simulink model "ECS_FOS"  (Simulink 8.2)
settings: Solver=ode45  StartTime=0.0  StopTime=18000  RelTol=1e-3
InitFcn:
  | load('loss_coeff_mixing_junction.mat')
  | load('SampleOutput.mat')
  | load('HydProp.mat')
  | load('HydraulicLoad.mat')
  | load('initavload.mat')
  | load('SampleFuelBurn.mat')
values from neighbouring files (symbols this model uses):
  FuelBurn = [0 0 0 0 0 0 0 0 0 0 0 0 ... (18249 elements, 1x18249)]    [Benchmark_data1.mat]
  fueltankdata =     [Benchmark_data1.mat]
undefined symbols (not defined in the file or in its folder): AirProp, F1, F2, HUGHES_TREITLER, magnitude, PN_70147, PumpProp
libraries: PowerFlowLib x46, simulink x4
(part 5 of 5)

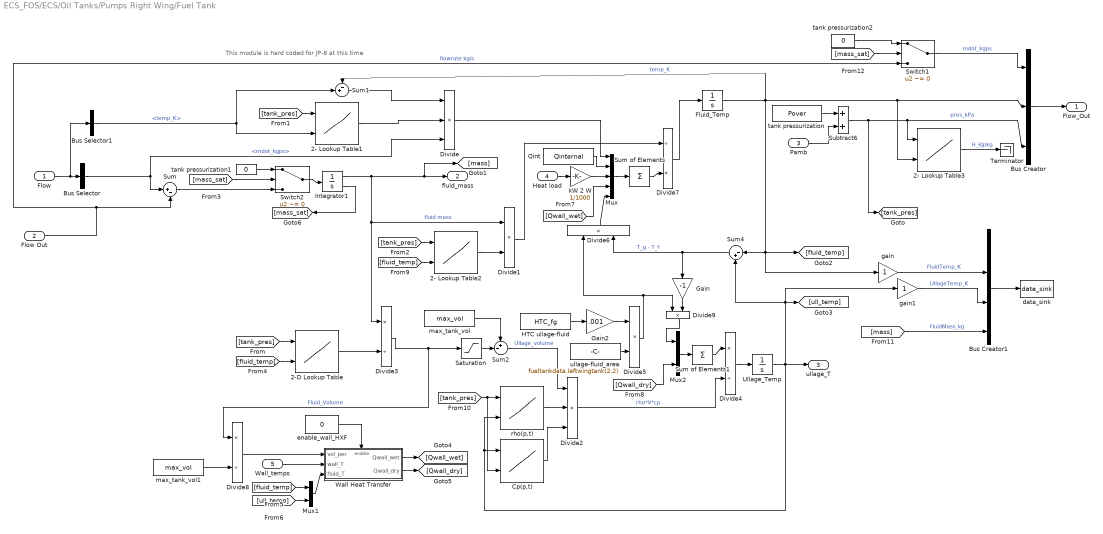
== system ECS_FOS/ECS/Oil Tanks/Pumps Right Wing/Fuel Tank ==
  note: This module is hard coded for JP-8 at this time
  Flow : Inport
  Flow Out : Inport  Port=2
  Pamb : Inport  Port=3
  Heat load : Inport  Port=4
  Wall_temps : Inport  Port=5
  2- Lookup Table1 : Lookup_n-D  BreakpointsForDimension1=F1.P  BreakpointsForDimension2=F1.T  Table=F1.Cp_pt  RndMeth=Simplest  InputSameDT=on
  2- Lookup Table2 : Lookup_n-D  BreakpointsForDimension1=F1.P  BreakpointsForDimension2=F1.T  Table=F1.Cp_pt  RndMeth=Simplest  InputSameDT=on
  2- Lookup Table3 : Lookup_n-D  BreakpointsForDimension1=F1.P  BreakpointsForDimension2=F1.T  Table=F1.H_pt  RndMeth=Simplest  InputSameDT=on
  2-D Lookup Table : Lookup_n-D  BreakpointsForDimension1=F1.P  BreakpointsForDimension2=F1.T  Table=F1.Rho_pt  RndMeth=Simplest  InputSameDT=on
  Bus Creator : BusCreator  Inputs=3
  Bus Creator1 : BusCreator
  Bus Selector : BusSelector  OutputSignals=mdot_kgps
  Bus Selector1 : BusSelector  OutputSignals=temp_K
  Cp(p,t) : Lookup_n-D  BreakpointsForDimension1=AirProp.P  BreakpointsForDimension2=AirProp.T  Table=AirProp.Cp_pt  RndMeth=Simplest  InputSameDT=on
  Divide : Product  Inputs=***
  Divide{1,5..6,9} (4 alike) : Product  Inputs=**
  Divide2 : Product  Inputs=***
  Divide3 : Product  Inputs=*/
  Divide4 : Product  Inputs=*/
  Divide7 : Product  Inputs=/*
  Divide8 : Product  Inputs=*/
  Fluid_Temp : Integrator  InitialCondition=fld_Tint + 273.15  LimitOutput=on  UpperSaturationLimit=800  LowerSaturationLimit=eps
  Gain : Gain  Gain=-1
  Gain2 : Gain  Gain=.001
  HTC ullage-fluid : Constant  Value=HTC_fg
  Integrator1 : Integrator  InitialCondition=m_init  LimitOutput=on  LowerSaturationLimit=1  ShowSaturationPort=on
  Mux : Mux  Inputs=5
  Mux1 : Mux  Inputs=2
  Mux2 : Mux  Inputs=2
  Qint : Constant  Value=Qinternal
  Saturation : Saturate  UpperLimit=inf  LowerLimit=eps  ZeroCross=off
  Subtract6 : Sum
  Sum : Sum  Inputs=|+-
  Sum of Elements : Sum  Inputs=+
  Sum of Elements1 : Sum  Inputs=+
  Sum1 : Sum  Inputs=-+|
  Sum2 : Sum  Inputs=+-|
  Sum4 : Sum  Inputs=|-+
  Switch1 : Switch  Criteria=u2 ~= 0  Threshold=-1
  Switch2 : Switch  Criteria=u2 ~= 0  Threshold=-1
  Terminator : Terminator
  Ullage_Temp : Integrator  InitialCondition=ull_Tint + 273.15  LimitOutput=on  LowerSaturationLimit=eps
  Wall Heat Transfer : Subsystem  TreatAsAtomicUnit=on
  data_sink : PowerFlowLib/Support Functions//Tools/data_sink
      link override global_data_goto: GotoTag=gdata_PowerFlowLibEnergyPowerSystemsThermalFuelFuelTank
  enable_wall_HXF : Constant  Value=0
  gain : Gain
  gain1 : Gain
  kW 2 W : Gain  Gain=1/1000
  max_tank_vol : Constant  Value=max_vol
  max_tank_vol1 : Constant  Value=max_vol
  rho(p,t) : Lookup_n-D  BreakpointsForDimension1=AirProp.P  BreakpointsForDimension2=AirProp.T  Table=AirProp.Rho_pt  RndMeth=Simplest  InputSameDT=on
  tank pressurization : Constant  Value=Pover
  tank pressurization1 : Constant  Value=0
  tank pressurization2 : Constant  Value=0
  ullage-fluid_area : Constant  Value=fueltankdata.leftwingtank(2,2)
  Flow_Out : Outport
  fluid_mass : Outport  Port=2
  ullage_T : Outport  Port=3
  wires:
  Switch2/1 -> Integrator1/1
  tank pressurization1/1 -> Switch2/1
  [mass_sat] -> Switch2/2
  Integrator1/2 -> [mass_sat]
  Sum/1 -> Switch2/3
  tank pressurization2/1 -> Switch1/1
  [mass_sat] -> Switch1/2
  [mass] -> Bus Creator1/4  "FluidMass_kg"
  gain1/1 -> Bus Creator1/3  "UllageTemp_K"
  gain/1 -> Bus Creator1/2  "FluidTemp_K"
  Bus Creator1/1 -> data_sink/1
  kW 2 W/1 -> Mux/3
  2- Lookup Table3/1 -> Terminator/1  "H_kJpkg"
  Flow/1 -> Bus Selector/1, Bus Selector1/1
  Bus Selector/1 -> Divide/3, Sum/1  "<mdot_kgps>"
  Flow Out/1 -> Sum/2, Switch1/3  "flowrate kg/s"
  Integrator1/1 -> fluid_mass/1, [mass], Divide3/1, Divide1/1  "fluid mass"
  Bus Selector1/1 -> Sum1/2, 2- Lookup Table1/2  "<temp_K>"
  Sum1/1 -> Divide/1
  2- Lookup Table2/1 -> Divide1/2
  rho(p,t)/1 -> Divide2/2
  Cp(p,t)/1 -> Divide2/3
  Divide3/1 -> Saturation/1, Divide8/1  "Fluid_Volume"
  max_tank_vol/1 -> Sum2/1
  Sum2/1 -> Divide2/1  "Ullage_volume"
  Divide4/1 -> Ullage_Temp/1
  Ullage_Temp/1 -> ullage_T/1, gain1/1, Sum4/2, [ull_temp], rho(p,t)/2, Cp(p,t)/1
  Fluid_Temp/1 -> 2- Lookup Table3/2, Bus Creator/2, Sum1/1, gain/1, Sum4/1, [fluid_temp]  "temp_K"
  HTC ullage-fluid/1 -> Gain2/1
  ullage-fluid_area/1 -> Divide5/2
  Sum4/1 -> Divide6/2, Gain/1  "T_g - T_f"
  Divide1/1 -> Divide7/1
  Divide7/1 -> Fluid_Temp/1
  Divide5/1 -> Divide6/1, Divide9/1
  Pamb/1 -> Subtract6/2
  tank pressurization/1 -> Subtract6/1
  Subtract6/1 -> 2- Lookup Table3/1, Bus Creator/3, [tank_pres]  "pres_kPa"
  Bus Creator/1 -> Flow_Out/1
  Saturation/1 -> Sum2/2
  [tank_pres] -> 2-D Lookup Table/1
  2-D Lookup Table/1 -> Divide3/2
  [tank_pres] -> 2- Lookup Table1/1
  2- Lookup Table1/1 -> Divide/2
  [tank_pres] -> 2- Lookup Table2/1
  max_tank_vol1/1 -> Divide8/2
  Switch1/1 -> Bus Creator/1  "mdot_kgps"
  Divide/1 -> Mux/1
  Qint/1 -> Mux/2
  Heat load/1 -> kW 2 W/1
  Sum of Elements/1 -> Divide7/2
  Mux/1 -> Sum of Elements/1
  [fluid_temp] -> 2-D Lookup Table/2
  Divide8/1 -> Wall Heat Transfer/1(vol_per)
  Wall_temps/1 -> Wall Heat Transfer/2(wall_T)
  [fluid_temp] -> Mux1/1
  [ull_temp] -> Mux1/2
  Mux1/1 -> Wall Heat Transfer/3(fluid_T)
  Wall Heat Transfer/1(Qwall_wet) -> [Qwall_wet]
  Wall Heat Transfer/2(Qwall_dry) -> [Qwall_dry]
  Divide6/1 -> Mux/5
  Divide2/1 -> Divide4/2  "rho*V*cp"
  Mux2/1 -> Sum of Elements1/1
  Sum of Elements1/1 -> Divide4/1
  Gain/1 -> Divide9/2
  Divide9/1 -> Mux2/1
  [Qwall_dry] -> Mux2/2
  [Qwall_wet] -> Mux/4
  [fluid_temp] -> 2- Lookup Table2/2
  enable_wall_HXF/1 -> Wall Heat Transfer/Enable
  Gain2/1 -> Divide5/1
  [tank_pres] -> rho(p,t)/1, Cp(p,t)/2

== system ECS_FOS/ECS/Right PACK/Distribution of bleed air ==
  Bleed to Valve : Inport
  Bleed to ACM : Inport  Port=2
  bleed_temp : Inport  Port=3
  bleed_pres : Inport  Port=4
  Bus Creator1 : BusCreator  Inputs=3
  Bus Creator2 : BusCreator  Inputs=3
  Scope : Scope  NumInputPorts=4
      settings: YMin=0~386.7~110~0.2  YMax=0.055~387.8~160~0.85  SaveName=ScopeData42  SampleInput=on  SampleTime=1
  Flow to Mix Junc. : Outport
  Flow to HX : Outport  Port=2
  wires:
  Bleed to ACM/1 -> Bus Creator2/1, Scope/4  "mdot_kgps"
  bleed_temp/1 -> Bus Creator2/2, Bus Creator1/2, Scope/2
  bleed_pres/1 -> Bus Creator2/3, Bus Creator1/3, Scope/3
  Bleed to Valve/1 -> Bus Creator1/1, Scope/1  "mdot_kgps"
  Bus Creator1/1 -> Flow to Mix Junc./1
  Bus Creator2/1 -> Flow to HX/1

== system ECS_FOS/ECS/Right PACK/Ram air inlet ==
  Temp_amb : Inport
  Temp_comp : Inport  Port=2
  2 : Constant  Value=T_35
  Bus Creator : BusCreator  Inputs=3
  Bus Selector4 : BusSelector  OutputSignals=temp_K
  Constant1 : Constant  Value=22.5
  Gain : Gain  Gain=0.95
  Gain1 : Gain
  Memory : Memory  X0=ram_air
  Subtract : Sum  Inputs=+-
  Switch : Switch  Criteria=u2 ~= 0  Threshold=30
  Flow Out : Outport
  wires:
  Temp_comp/1 -> Bus Selector4/1
  Bus Selector4/1 -> Subtract/1  "<temp_K>"
  2/1 -> Subtract/2
  Subtract/1 -> Switch/2
  Gain/1 -> Switch/3
  Switch/1 -> Memory/1
  Temp_amb/1 -> Bus Creator/1  "temp_K"
  Constant1/1 -> Bus Creator/2  "pres_kPa"
  Bus Creator/1 -> Flow Out/1
  Memory/1 -> Bus Creator/3, Gain1/1, Gain/1  "mdot_kgps"
  Gain1/1 -> Switch/1

== system ECS_FOS/ECS/Right PACK/Subsystem1 ==
  Bypass Ratio : Inport
  Air from PHX : Inport  Port=2
  Bus Creator : BusCreator  Inputs=3
  Bus Creator1 : BusCreator  Inputs=3
  Bus Selector : BusSelector  OutputSignals=mdot_kgps,temp_K,pres_kPa
  Fcn1 : Fcn  Expr=1-u(1)
  Gain : Gain
  Gain1 : Gain
  Gain2 : Gain
  Product : Product  RndMeth=Zero
  Product1 : Product  RndMeth=Zero
  Saturation : Saturate  UpperLimit=inf  LowerLimit=eps
  Air to Mix Junc : Outport
  Air to Comp : Outport  Port=2
  wires:
  Gain1/1 -> Bus Creator1/2  "temp_K"
  Gain/1 -> Bus Creator1/3  "pres_kPa"
  Bus Creator1/1 -> Air to Mix Junc/1
  Bus Selector/3 -> Gain/1, Gain2/1  "<pres_kPa>"
  Product1/1 -> Bus Creator1/1  "mdot_kgps"
  Saturation/1 -> Bus Creator/1  "mdot_kgps"
  Bus Selector/2 -> Gain1/1, Bus Creator/2  "<temp_K>"
  Bus Creator/1 -> Air to Comp/1
  Bus Selector/1 -> Product/2, Product1/1  "<mdot_kgps>"
  Air from PHX/1 -> Bus Selector/1
  Product/1 -> Saturation/1
  Bypass Ratio/1 -> Fcn1/1, Product1/2
  Fcn1/1 -> Product/1
  Gain2/1 -> Bus Creator/3  "pres_kPa"

== system ECS_FOS/ECS/Right PACK/User-set_ supply_pressure ==
  Flow In : Inport
  Cabin Pres. : Inport  Port=2
  Bus Creator4 : BusCreator  Inputs=3
  Bus Selector3 : BusSelector  OutputSignals=mdot_kgps,temp_K
  Gain1 : Gain  Gain=1.1
  Flow Out : Outport
  wires:
  Bus Selector3/1 -> Bus Creator4/1  "<mdot_kgps>"
  Bus Selector3/2 -> Bus Creator4/2  "<temp_K>"
  Gain1/1 -> Bus Creator4/3  "pres_kPa"
  Flow In/1 -> Bus Selector3/1
  Bus Creator4/1 -> Flow Out/1
  Cabin Pres./1 -> Gain1/1

== system ECS_FOS/ECS/Right PACK/Valve1 ==
  Flow In : Inport
  Bus Creator2 : BusCreator  Inputs=3
  Bus Selector2 : BusSelector  OutputSignals=mdot_kgps,pres_kPa,temp_K
  Math Functin : Math  Operator=pow  SaturateOnIntegerOverflow=on
  Product : Product  RndMeth=Zero
  Sum : Sum  Inputs=|-+
  "Value?? -- MAW" : Constant  Value=50
  get u : Gain
  mass_flow_rate1 : Constant  Value=2
  Flow Out : Outport
  wires:
  Bus Creator2/1 -> Flow Out/1
  Flow In/1 -> Bus Selector2/1
  Bus Selector2/1 -> Bus Creator2/1, get u/1  "<mdot_kgps>"
  get u/1 -> Math Functin/1
  mass_flow_rate1/1 -> Math Functin/2
  Math Functin/1 -> Product/2
  Product/1 -> Sum/1
  Bus Selector2/2 -> Sum/2  "<pres_kPa>"
  Sum/1 -> Bus Creator2/2  "pres_kPa"
  Bus Selector2/3 -> Bus Creator2/3  "<temp_K>"
  "Value?? -- MAW"/1 -> Product/1

== system ECS_FOS/ECS/Thermal_sources_from Electrical_power_model1/ThermalSource ==
  LoadBus : BusCreator  Inputs=1
  Load : Outport
  wires:
  LoadBus/1 -> Load/1

== system ECS_FOS/ECS/Thermal_sources_from Electrical_power_model1/ThermalSource3 ==
  LoadBus : BusCreator  Inputs=1
  Load : Outport
  wires:
  LoadBus/1 -> Load/1

== system ECS_FOS/ECS/Thermal_sources_from Electrical_power_model1/ThermalSource4 ==
  LoadBus : BusCreator  Inputs=1
  Load : Outport
  wires:
  LoadBus/1 -> Load/1

== system ECS_FOS/ECS/Thermal_sources_from Electrical_power_model1/ThermalSource5 ==
  LoadBus : BusCreator  Inputs=1
  Load : Outport
  wires:
  LoadBus/1 -> Load/1

== system ECS_FOS/ECS/Cabin Zone/Cabin Temperature/Fuselage_parameters1 ==
  Area_fuselage_total_m2 : Constant  Value=A_fuselage
  Bus Creator : BusCreator  Inputs=2
  Coating_resistance_ m2KpW : Product  Inputs=*/
  Coating_thermal_ conductivity_WpmK : Constant  Value=K_coating
  Coating_thickness_m : Constant  Value=L_coating
  Display : Display
  Inside_HTC_Wpm2K : Constant  Value=h_inside
  Inside_convection_ resistance_m2KpW : Product  Inputs=*/
  Insulation_resistance_ m2KpW : Product  Inputs=*/
  Insulation_thermal_ conductivity_WpmK : Constant  Value=K_insulation
  Insulation_thickness_m : Constant  Value=L_insulation
  Outside_HTC_Wpm2K1 : Constant  Value=h_outside
  Outside_convection_ resistance_m2KpW : Product  Inputs=*/
  Overall_HTC_based_on_ any_fuselage_area_Wpm2K : Product  Inputs=*/
  Shell_resistance_ m2KpW : Product  Inputs=*/
  Shell_thermal_ conductivity_WpmK : Constant  Value=K_shell
  Shell_thickness_m : Constant  Value=L_shell
  Total_resistance_ m2KpW : Sum  Inputs=+++++
  constant_unity : Constant
  constant_unity1 : Constant
  constant_unity2 : Constant
  Fuselage Parameters : Outport
  wires:
  Overall_HTC_based_on_ any_fuselage_area_Wpm2K/1 -> Bus Creator/2, Display/1  "U_Wpm2K"
  Bus Creator/1 -> Fuselage Parameters/1
  constant_unity/1 -> Outside_convection_ resistance_m2KpW/1
  Outside_HTC_Wpm2K1/1 -> Outside_convection_ resistance_m2KpW/2
  Shell_thickness_m/1 -> Shell_resistance_ m2KpW/1
  Shell_thermal_ conductivity_WpmK/1 -> Shell_resistance_ m2KpW/2
  Insulation_thickness_m/1 -> Insulation_resistance_ m2KpW/1
  Insulation_thermal_ conductivity_WpmK/1 -> Insulation_resistance_ m2KpW/2
  Coating_thickness_m/1 -> Coating_resistance_ m2KpW/1
  Coating_thermal_ conductivity_WpmK/1 -> Coating_resistance_ m2KpW/2
  constant_unity1/1 -> Inside_convection_ resistance_m2KpW/1
  Inside_HTC_Wpm2K/1 -> Inside_convection_ resistance_m2KpW/2
  Outside_convection_ resistance_m2KpW/1 -> Total_resistance_ m2KpW/1
  Shell_resistance_ m2KpW/1 -> Total_resistance_ m2KpW/2
  Insulation_resistance_ m2KpW/1 -> Total_resistance_ m2KpW/3
  Coating_resistance_ m2KpW/1 -> Total_resistance_ m2KpW/4
  Inside_convection_ resistance_m2KpW/1 -> Total_resistance_ m2KpW/5
  constant_unity2/1 -> Overall_HTC_based_on_ any_fuselage_area_Wpm2K/1
  Total_resistance_ m2KpW/1 -> Overall_HTC_based_on_ any_fuselage_area_Wpm2K/2
  Area_fuselage_total_m2/1 -> Bus Creator/1  "area_m2"

== system ECS_FOS/ECS/Cabin Zone/Cabin Temperature/Kinetic Heating ==
  note: PLEASE note that that the correlation for the recovery temperature
      | is gives in "Aircraft Systems", by Ian Moir and Allan Seabridge,
      | 3rd edition, pp 260
  Amb. Temp. K : Inport
  Mach# : Inport  Port=2
  Bias : Bias  Bias=1
  Gain : Gain  Gain=0.18
  Math Function1 : Math  Operator=magnitude^2  SaturateOnIntegerOverflow=on
  Product1 : Product  RndMeth=Zero
  Recovery Temp [K] : Outport
  wires:
  Mach#/1 -> Math Function1/1
  Product1/1 -> Recovery Temp [K]/1
  Amb. Temp. K/1 -> Product1/1
  Bias/1 -> Product1/2
  Gain/1 -> Bias/1
  Math Function1/1 -> Gain/1

== system ECS_FOS/ECS/FOHX Left Wing/HX_Calcs/Fluid 1 Heat Transfer Calculation ==
  note: NTU calculation
  note: Secondary Fluid heat transfer coefficient
  note: It calculates the outlet temperature and enthalpy.
  Inputs : Inport
  2-D Lookup Table : Lookup_n-D  BreakpointsForDimension1=F1.P  BreakpointsForDimension2=F1.T  Table=F1.H_pt  RndMeth=Simplest  InputSameDT=on
  2-D Lookup Table1 : Lookup_n-D  BreakpointsForDimension1=F1.P  BreakpointsForDimension2=F1.T  Table=F1.H_pt  RndMeth=Simplest  InputSameDT=on
  2-D Lookup Table2 : Lookup_n-D  BreakpointsForDimension1=F1.P  BreakpointsForDimension2=F1.T  Table=F1.H_pt  RndMeth=Simplest  InputSameDT=on
  2-D Lookup Table3 : Lookup_n-D  BreakpointsForDimension1=F1.P  BreakpointsForDimension2=F1.T  Table=F1.Cp_pt  RndMeth=Simplest  InputSameDT=on
  Bus Selector : BusSelector  OutputSignals=mdot1_in,T1_in,P1_in
  Constant : Constant  Value=0
  Constant10 : Constant  Value=A1_c
  Constant2 : Constant  Value=N1
  Constant4 : Constant
  Constant8 : Constant  Value=N1
  Constant9 : Constant  Value=A1_s*2
  Fcn6 : Fcn  Expr=u(2) + (u(1)-u(2))*u(3)
  Gain1 : Gain  Gain=-1
  Gain3 : Gain
  HTC Calc : Subsystem
  Math Function3 : Math  SaturateOnIntegerOverflow=on
  Mux4 : Mux  Inputs=3
  Product2 : Product  Inputs=***//  RndMeth=Zero
  Product6 : Product  Inputs=***/  RndMeth=Zero
  Subtract2 : Sum  Inputs=+-
  kJ/kg to J/kg : Gain  Gain=1000
  h_out_h : Outport
  T_out_h : Outport  Port=2
  q_h : Outport  Port=3
  wires:
  [T_out] -> 2-D Lookup Table1/2
  [T_in] -> 2-D Lookup Table/2
  2-D Lookup Table/1 -> Subtract2/1
  2-D Lookup Table1/1 -> Subtract2/2
  2-D Lookup Table2/1 -> h_out_h/1
  Product6/1 -> Gain1/1
  Constant4/1 -> Product6/2
  [mdot_in] -> Product6/1
  Subtract2/1 -> Product6/3
  Fcn6/1 -> T_out_h/1, [T_out], 2-D Lookup Table2/2  "T_out"
  Mux4/1 -> Fcn6/1
  [e2NTU1] -> Mux4/3
  Constant/1 -> Mux4/2
  Gain1/1 -> q_h/1
  Constant2/1 -> Product6/4
  Product2/1 -> Gain3/1  "NTU"
  Constant9/1 -> Product2/2
  [alpha] -> Product2/1
  Constant8/1 -> Product2/3
  HTC Calc/1(alpha_a) -> [alpha]
  [T_in] -> HTC Calc/3(T_a)
  Constant10/1 -> HTC Calc/2(A_ca)
  [mdot_in] -> HTC Calc/1(mdot_a)
  [T_in] -> 2-D Lookup Table3/2
  2-D Lookup Table3/1 -> kJ/kg to J/kg/1
  Inputs/1 -> Bus Selector/1
  Bus Selector/1 -> [mdot_in]  "<mdot1_in>"
  Bus Selector/2 -> [T_in]  "<T1_in>"
  Bus Selector/3 -> [P_in]  "<P1_in>"
  Math Function3/1 -> [e2NTU1]
  Gain3/1 -> Math Function3/1
  [mdot_in] -> Product2/4
  [cp] -> Product2/5
  [T_in] -> Mux4/1
  [P_in] -> 2-D Lookup Table/1
  [P_in] -> 2-D Lookup Table1/1
  [P_in] -> 2-D Lookup Table2/1
  [P_in] -> 2-D Lookup Table3/1
  kJ/kg to J/kg/1 -> [cp]

== system ECS_FOS/ECS/FOHX Left Wing/HX_Calcs/Fluid 2 Heat Transfer Calculation ==
  note: NTU calculation
  note: Secondary Fluid heat transfer coefficient
  note: It calculates the outlet temperature and enthalpy.
  Inputs : Inport
  1-D Lookup Table : Lookup_n-D  NumberOfTableDimensions=1  BreakpointsForDimension1=F2.T  Table=F2.cp_T  RndMeth=Simplest  InputSameDT=on
  1-D Lookup Table1 : Lookup_n-D  NumberOfTableDimensions=1  BreakpointsForDimension1=F2.T  Table=F2.H  RndMeth=Simplest  InputSameDT=on
  1-D Lookup Table2 : Lookup_n-D  NumberOfTableDimensions=1  BreakpointsForDimension1=F2.T  Table=F2.H  RndMeth=Simplest  InputSameDT=on
  1-D Lookup Table3 : Lookup_n-D  NumberOfTableDimensions=1  BreakpointsForDimension1=F2.T  Table=F2.H  RndMeth=Simplest  InputSameDT=on
  Bus Selector : BusSelector  OutputSignals=mdot2_in,T2_in,P2_in
  Constant : Constant  Value=0
  Constant10 : Constant  Value=A2_c
  Constant2 : Constant  Value=N2
  Constant4 : Constant
  Constant8 : Constant  Value=N2
  Constant9 : Constant  Value=A2_s*2
  Fcn6 : Fcn  Expr=u(2) + (u(1)-u(2))*u(3)
  Gain1 : Gain  Gain=-1
  Gain3 : Gain  Gain=-1
  HTC Calc : Subsystem
  Math Function3 : Math  SaturateOnIntegerOverflow=on
  Mux4 : Mux  Inputs=3
  Product2 : Product  Inputs=***//  RndMeth=Zero
  Product6 : Product  Inputs=***/  RndMeth=Zero
  Subtract2 : Sum  Inputs=+-
  Terminator : Terminator
  kJ/kg to J/kg : Gain  Gain=1000
  h_out : Outport
  T_out : Outport  Port=2
  q_h : Outport  Port=3
  wires:
  [T_out] -> 1-D Lookup Table3/1
  [T_in] -> 1-D Lookup Table2/1
  1-D Lookup Table2/1 -> Subtract2/1
  1-D Lookup Table3/1 -> Subtract2/2
  1-D Lookup Table1/1 -> h_out/1
  Product6/1 -> Gain1/1
  Constant4/1 -> Product6/2
  [mdot_in] -> Product6/1
  Subtract2/1 -> Product6/3
  Fcn6/1 -> [T_out], T_out/1, 1-D Lookup Table1/1  "T_out"
  Mux4/1 -> Fcn6/1
  [e2NTU1] -> Mux4/3
  Constant/1 -> Mux4/2
  Gain1/1 -> q_h/1
  Constant2/1 -> Product6/4
  Product2/1 -> Gain3/1  "NTU"
  Constant9/1 -> Product2/2
  [alpha] -> Product2/1
  Constant8/1 -> Product2/3
  HTC Calc/1(alpha_a) -> [alpha]
  [T_in] -> HTC Calc/3(T_a)
  Constant10/1 -> HTC Calc/2(A_ca)
  [mdot_in] -> HTC Calc/1(mdot_a)
  [T_in] -> 1-D Lookup Table/1
  1-D Lookup Table/1 -> kJ/kg to J/kg/1
  Inputs/1 -> Bus Selector/1
  Bus Selector/1 -> [mdot_in]  "<mdot2_in>"
  Bus Selector/2 -> [T_in]  "<T2_in>"
  Bus Selector/3 -> Terminator/1  "<P2_in>"
  Math Function3/1 -> [e2NTU1]
  Gain3/1 -> Math Function3/1
  [mdot_in] -> Product2/4
  [cp] -> Product2/5
  [T_in] -> Mux4/1
  kJ/kg to J/kg/1 -> [cp]

== system ECS_FOS/ECS/FOHX Left Wing/HX_Calcs/Input Processing ==
  Inputs : Inport
  Bus Creator : BusCreator  Inputs=6
  Bus Selector : BusSelector  OutputSignals=mdot1_in,P1_in,T1_in,mdot2_in,P2_in,T2_in
  Processed_Inputs : Outport
  wires:
  Bus Selector/1 -> Bus Creator/1  "<mdot1_in>"
  Bus Selector/2 -> Bus Creator/2  "<P1_in>"
  Bus Selector/3 -> Bus Creator/3  "<T1_in>"
  Bus Selector/4 -> Bus Creator/4  "<mdot2_in>"
  Bus Selector/5 -> Bus Creator/5  "<P2_in>"
  Bus Selector/6 -> Bus Creator/6  "<T2_in>"
  Inputs/1 -> Bus Selector/1  "Inputs"
  Bus Creator/1 -> Processed_Inputs/1

== system ECS_FOS/ECS/FOHX Right Wing/HX_Calcs/Fluid 1 Heat Transfer Calculation ==
  note: It calculates the outlet temperature and enthalpy.
  note: Secondary Fluid heat transfer coefficient
  note: NTU calculation
  Inputs : Inport
  2-D Lookup Table : Lookup_n-D  BreakpointsForDimension1=F1.P  BreakpointsForDimension2=F1.T  Table=F1.H_pt  RndMeth=Simplest  InputSameDT=on
  2-D Lookup Table1 : Lookup_n-D  BreakpointsForDimension1=F1.P  BreakpointsForDimension2=F1.T  Table=F1.H_pt  RndMeth=Simplest  InputSameDT=on
  2-D Lookup Table2 : Lookup_n-D  BreakpointsForDimension1=F1.P  BreakpointsForDimension2=F1.T  Table=F1.H_pt  RndMeth=Simplest  InputSameDT=on
  2-D Lookup Table3 : Lookup_n-D  BreakpointsForDimension1=F1.P  BreakpointsForDimension2=F1.T  Table=F1.Cp_pt  RndMeth=Simplest  InputSameDT=on
  Bus Selector : BusSelector  OutputSignals=mdot1_in,T1_in,P1_in
  Constant : Constant  Value=0
  Constant10 : Constant  Value=A1_c
  Constant2 : Constant  Value=N1
  Constant4 : Constant
  Constant8 : Constant  Value=N1
  Constant9 : Constant  Value=A1_s*2
  Fcn6 : Fcn  Expr=u(2) + (u(1)-u(2))*u(3)
  Gain1 : Gain  Gain=-1
  Gain3 : Gain
  HTC Calc : Subsystem
  Math Function3 : Math  SaturateOnIntegerOverflow=on
  Mux4 : Mux  Inputs=3
  Product2 : Product  Inputs=***//  RndMeth=Zero
  Product6 : Product  Inputs=***/  RndMeth=Zero
  Subtract2 : Sum  Inputs=+-
  kJ/kg to J/kg : Gain  Gain=1000
  h_out_h : Outport
  T_out_h : Outport  Port=2
  q_h : Outport  Port=3
  wires:
  kJ/kg to J/kg/1 -> [cp]
  [P_in] -> 2-D Lookup Table3/1
  [P_in] -> 2-D Lookup Table2/1
  [P_in] -> 2-D Lookup Table1/1
  [P_in] -> 2-D Lookup Table/1
  [T_in] -> Mux4/1
  [cp] -> Product2/5
  [mdot_in] -> Product2/4
  Gain3/1 -> Math Function3/1
  Math Function3/1 -> [e2NTU1]
  Bus Selector/3 -> [P_in]  "<P1_in>"
  Bus Selector/2 -> [T_in]  "<T1_in>"
  Bus Selector/1 -> [mdot_in]  "<mdot1_in>"
  Inputs/1 -> Bus Selector/1
  2-D Lookup Table3/1 -> kJ/kg to J/kg/1
  [T_in] -> 2-D Lookup Table3/2
  [mdot_in] -> HTC Calc/1(mdot_a)
  Constant10/1 -> HTC Calc/2(A_ca)
  [T_in] -> HTC Calc/3(T_a)
  HTC Calc/1(alpha_a) -> [alpha]
  Constant8/1 -> Product2/3
  [alpha] -> Product2/1
  Constant9/1 -> Product2/2
  Product2/1 -> Gain3/1  "NTU"
  Constant2/1 -> Product6/4
  Gain1/1 -> q_h/1
  Constant/1 -> Mux4/2
  [e2NTU1] -> Mux4/3
  Mux4/1 -> Fcn6/1
  Fcn6/1 -> 2-D Lookup Table2/2, [T_out], T_out_h/1  "T_out"
  Subtract2/1 -> Product6/3
  [mdot_in] -> Product6/1
  Constant4/1 -> Product6/2
  Product6/1 -> Gain1/1
  2-D Lookup Table2/1 -> h_out_h/1
  2-D Lookup Table1/1 -> Subtract2/2
  2-D Lookup Table/1 -> Subtract2/1
  [T_in] -> 2-D Lookup Table/2
  [T_out] -> 2-D Lookup Table1/2

== system ECS_FOS/ECS/FOHX Right Wing/HX_Calcs/Fluid 2 Heat Transfer Calculation ==
  note: It calculates the outlet temperature and enthalpy.
  note: Secondary Fluid heat transfer coefficient
  note: NTU calculation
  Inputs : Inport
  1-D Lookup Table : Lookup_n-D  NumberOfTableDimensions=1  BreakpointsForDimension1=F2.T  Table=F2.cp_T  RndMeth=Simplest  InputSameDT=on
  1-D Lookup Table1 : Lookup_n-D  NumberOfTableDimensions=1  BreakpointsForDimension1=F2.T  Table=F2.H  RndMeth=Simplest  InputSameDT=on
  1-D Lookup Table2 : Lookup_n-D  NumberOfTableDimensions=1  BreakpointsForDimension1=F2.T  Table=F2.H  RndMeth=Simplest  InputSameDT=on
  1-D Lookup Table3 : Lookup_n-D  NumberOfTableDimensions=1  BreakpointsForDimension1=F2.T  Table=F2.H  RndMeth=Simplest  InputSameDT=on
  Bus Selector : BusSelector  OutputSignals=mdot2_in,T2_in,P2_in
  Constant : Constant  Value=0
  Constant10 : Constant  Value=A2_c
  Constant2 : Constant  Value=N2
  Constant4 : Constant
  Constant8 : Constant  Value=N2
  Constant9 : Constant  Value=A2_s*2
  Fcn6 : Fcn  Expr=u(2) + (u(1)-u(2))*u(3)
  Gain1 : Gain  Gain=-1
  Gain3 : Gain  Gain=-1
  HTC Calc : Subsystem
  Math Function3 : Math  SaturateOnIntegerOverflow=on
  Mux4 : Mux  Inputs=3
  Product2 : Product  Inputs=***//  RndMeth=Zero
  Product6 : Product  Inputs=***/  RndMeth=Zero
  Subtract2 : Sum  Inputs=+-
  Terminator : Terminator
  kJ/kg to J/kg : Gain  Gain=1000
  h_out : Outport
  T_out : Outport  Port=2
  q_h : Outport  Port=3
  wires:
  kJ/kg to J/kg/1 -> [cp]
  [T_in] -> Mux4/1
  [cp] -> Product2/5
  [mdot_in] -> Product2/4
  Gain3/1 -> Math Function3/1
  Math Function3/1 -> [e2NTU1]
  Bus Selector/3 -> Terminator/1  "<P2_in>"
  Bus Selector/2 -> [T_in]  "<T2_in>"
  Bus Selector/1 -> [mdot_in]  "<mdot2_in>"
  Inputs/1 -> Bus Selector/1
  1-D Lookup Table/1 -> kJ/kg to J/kg/1
  [T_in] -> 1-D Lookup Table/1
  [mdot_in] -> HTC Calc/1(mdot_a)
  Constant10/1 -> HTC Calc/2(A_ca)
  [T_in] -> HTC Calc/3(T_a)
  HTC Calc/1(alpha_a) -> [alpha]
  Constant8/1 -> Product2/3
  [alpha] -> Product2/1
  Constant9/1 -> Product2/2
  Product2/1 -> Gain3/1  "NTU"
  Constant2/1 -> Product6/4
  Gain1/1 -> q_h/1
  Constant/1 -> Mux4/2
  [e2NTU1] -> Mux4/3
  Mux4/1 -> Fcn6/1
  Fcn6/1 -> 1-D Lookup Table1/1, T_out/1, [T_out]  "T_out"
  Subtract2/1 -> Product6/3
  [mdot_in] -> Product6/1
  Constant4/1 -> Product6/2
  Product6/1 -> Gain1/1
  1-D Lookup Table1/1 -> h_out/1
  1-D Lookup Table3/1 -> Subtract2/2
  1-D Lookup Table2/1 -> Subtract2/1
  [T_in] -> 1-D Lookup Table2/1
  [T_out] -> 1-D Lookup Table3/1

== system ECS_FOS/ECS/FOHX Right Wing/HX_Calcs/Input Processing ==
  Inputs : Inport
  Bus Creator : BusCreator  Inputs=6
  Bus Selector : BusSelector  OutputSignals=mdot1_in,P1_in,T1_in,mdot2_in,P2_in,T2_in
  Processed_Inputs : Outport
  wires:
  Bus Creator/1 -> Processed_Inputs/1
  Inputs/1 -> Bus Selector/1  "Inputs"
  Bus Selector/6 -> Bus Creator/6  "<T2_in>"
  Bus Selector/5 -> Bus Creator/5  "<P2_in>"
  Bus Selector/4 -> Bus Creator/4  "<mdot2_in>"
  Bus Selector/3 -> Bus Creator/3  "<T1_in>"
  Bus Selector/2 -> Bus Creator/2  "<P1_in>"
  Bus Selector/1 -> Bus Creator/1  "<mdot1_in>"

== system ECS_FOS/ECS/Fuel Tanks/Pumps/Center Fuel Tank/Wall Heat Transfer ==
  vol_per : Inport
  wall_T : Inport  Port=2
  fluid_T : Inport  Port=3
  Enable : EnablePort
  Abs : Abs
  Demux : Demux  Outputs=2
  Divide : Product  Inputs=**
  Divide1 : Product  Inputs=**
  Sum : Sum  Inputs=+-
  Sum1 : Sum  Inputs=-+
  Walls 1 to n : Constant  Value=1:size(fueltankdata.centertank,2)
  dry HTC : Gain  Gain=dryHTC
  total area : Bias  Bias=-[fueltankdata.centertank(11,:)]
  volume_% : Lookup_n-D  BreakpointsForDimension1=linspace(0,1,11)  BreakpointsForDimension2=linspace(1,6,6)  Table=fueltankdata.centertank  RndMeth=Simplest  InputSameDT=on
  wet HTC : Gain  Gain=wetHTC
  Qwall_wet : Outport
  Qwall_dry : Outport  Port=2
  wires:
  Walls 1 to n/1 -> volume_%/2
  vol_per/1 -> volume_%/1
  volume_%/1 -> total area/1, wet HTC/1  "wet area"
  fluid_T/1 -> Demux/1
  Demux/1 -> Sum/2  "fuel temp"
  Demux/2 -> Sum1/1  "ullage temp"
  wall_T/1 -> Sum/1, Sum1/2
  Sum/1 -> Divide/2  "T_wall - T_fuel"
  Sum1/1 -> Divide1/2  "T_wall - T_ull"
  wet HTC/1 -> Divide/1
  total area/1 -> Abs/1  "dry area"
  Divide/1 -> Qwall_wet/1
  Divide1/1 -> Qwall_dry/1
  dry HTC/1 -> Divide1/1
  Abs/1 -> dry HTC/1

== system ECS_FOS/ECS/Fuel Tanks/Pumps/Left Wing Fuel Tank/Wall Heat Transfer ==
  vol_per : Inport
  wall_T : Inport  Port=2
  fluid_T : Inport  Port=3
  Enable : EnablePort
  Abs : Abs
  Demux : Demux  Outputs=2
  Divide : Product  Inputs=**
  Divide1 : Product  Inputs=**
  Sum : Sum  Inputs=+-
  Sum1 : Sum  Inputs=-+
  Walls 1 to n : Constant  Value=1:size(fueltankdata.leftwingtank,2)
  dry HTC : Gain  Gain=dryHTC
  total area : Bias  Bias=-[fueltankdata.leftwingtank(11,:)]
  volume_% : Lookup_n-D  BreakpointsForDimension1=linspace(0,1,11)  BreakpointsForDimension2=linspace(1,6,6)  Table=fueltankdata.leftwingtank  RndMeth=Simplest  InputSameDT=on
  wet HTC : Gain  Gain=wetHTC
  Qwall_wet : Outport
  Qwall_dry : Outport  Port=2
  wires:
  Walls 1 to n/1 -> volume_%/2
  vol_per/1 -> volume_%/1
  volume_%/1 -> total area/1, wet HTC/1  "wet area"
  fluid_T/1 -> Demux/1
  Demux/1 -> Sum/2  "fuel temp"
  Demux/2 -> Sum1/1  "ullage temp"
  wall_T/1 -> Sum/1, Sum1/2
  Sum/1 -> Divide/2  "T_wall - T_fuel"
  Sum1/1 -> Divide1/2  "T_wall - T_ull"
  wet HTC/1 -> Divide/1
  total area/1 -> Abs/1  "dry area"
  Divide/1 -> Qwall_wet/1
  Divide1/1 -> Qwall_dry/1
  dry HTC/1 -> Divide1/1
  Abs/1 -> dry HTC/1

== system ECS_FOS/ECS/Fuel Tanks/Pumps/Right Wing Fuel Tank/Wall Heat Transfer ==
  vol_per : Inport
  wall_T : Inport  Port=2
  fluid_T : Inport  Port=3
  Enable : EnablePort
  Abs : Abs
  Demux : Demux  Outputs=2
  Divide : Product  Inputs=**
  Divide1 : Product  Inputs=**
  Sum : Sum  Inputs=+-
  Sum1 : Sum  Inputs=-+
  Walls 1 to n : Constant  Value=1:size(fueltankdata.rightwingtank,2)
  dry HTC : Gain  Gain=dryHTC
  total area : Bias  Bias=-[fueltankdata.rightwingtank(11,:)]
  volume_% : Lookup_n-D  BreakpointsForDimension1=linspace(0,1,11)  BreakpointsForDimension2=linspace(1,6,6)  Table=fueltankdata.rightwingtank  RndMeth=Simplest  InputSameDT=on
  wet HTC : Gain  Gain=wetHTC
  Qwall_wet : Outport
  Qwall_dry : Outport  Port=2
  wires:
  Walls 1 to n/1 -> volume_%/2
  vol_per/1 -> volume_%/1
  volume_%/1 -> total area/1, wet HTC/1  "wet area"
  fluid_T/1 -> Demux/1
  Demux/1 -> Sum/2  "fuel temp"
  Demux/2 -> Sum1/1  "ullage temp"
  wall_T/1 -> Sum/1, Sum1/2
  Sum/1 -> Divide/2  "T_wall - T_fuel"
  Sum1/1 -> Divide1/2  "T_wall - T_ull"
  wet HTC/1 -> Divide/1
  total area/1 -> Abs/1  "dry area"
  Divide/1 -> Qwall_wet/1
  Divide1/1 -> Qwall_dry/1
  dry HTC/1 -> Divide1/1
  Abs/1 -> dry HTC/1

== system ECS_FOS/ECS/Oil Tanks/Pumps Left Wing/Oil Tank/Wall Heat Transfer ==
  vol_per : Inport
  wall_T : Inport  Port=2
  fluid_T : Inport  Port=3
  Enable : EnablePort
  Abs : Abs
  Demux : Demux  Outputs=2
  Divide : Product  Inputs=**
  Divide1 : Product  Inputs=**
  Sum : Sum  Inputs=+-
  Sum1 : Sum  Inputs=-+
  Walls 1 to n : Constant  Value=1:size(fueltankdata.leftwingtank,2)
  dry HTC : Gain  Gain=dryHTC
  total area : Bias  Bias=-[fueltankdata.leftwingtank(11,:)]
  volume_% : Lookup_n-D  BreakpointsForDimension1=linspace(0,1,11)  BreakpointsForDimension2=linspace(1,6,6)  Table=fueltankdata.leftwingtank  RndMeth=Simplest  InputSameDT=on
  wet HTC : Gain  Gain=wetHTC
  Qwall_wet : Outport
  Qwall_dry : Outport  Port=2
  wires:
  Walls 1 to n/1 -> volume_%/2
  vol_per/1 -> volume_%/1
  volume_%/1 -> total area/1, wet HTC/1  "wet area"
  fluid_T/1 -> Demux/1
  Demux/1 -> Sum/2  "fuel temp"
  Demux/2 -> Sum1/1  "ullage temp"
  wall_T/1 -> Sum/1, Sum1/2
  Sum/1 -> Divide/2  "T_wall - T_fuel"
  Sum1/1 -> Divide1/2  "T_wall - T_ull"
  wet HTC/1 -> Divide/1
  total area/1 -> Abs/1  "dry area"
  Divide/1 -> Qwall_wet/1
  Divide1/1 -> Qwall_dry/1
  dry HTC/1 -> Divide1/1
  Abs/1 -> dry HTC/1

== system ECS_FOS/ECS/Oil Tanks/Pumps Right Wing/Fuel Tank/Wall Heat Transfer ==
  vol_per : Inport
  wall_T : Inport  Port=2
  fluid_T : Inport  Port=3
  Enable : EnablePort
  Abs : Abs
  Demux : Demux  Outputs=2
  Divide : Product  Inputs=**
  Divide1 : Product  Inputs=**
  Sum : Sum  Inputs=+-
  Sum1 : Sum  Inputs=-+
  Walls 1 to n : Constant  Value=1:size(fueltankdata.leftwingtank,2)
  dry HTC : Gain  Gain=dryHTC
  total area : Bias  Bias=-[fueltankdata.leftwingtank(11,:)]
  volume_% : Lookup_n-D  BreakpointsForDimension1=linspace(0,1,11)  BreakpointsForDimension2=linspace(1,6,6)  Table=fueltankdata.leftwingtank  RndMeth=Simplest  InputSameDT=on
  wet HTC : Gain  Gain=wetHTC
  Qwall_wet : Outport
  Qwall_dry : Outport  Port=2
  wires:
  Walls 1 to n/1 -> volume_%/2
  vol_per/1 -> volume_%/1
  volume_%/1 -> total area/1, wet HTC/1  "wet area"
  fluid_T/1 -> Demux/1
  Demux/1 -> Sum/2  "fuel temp"
  Demux/2 -> Sum1/1  "ullage temp"
  wall_T/1 -> Sum/1, Sum1/2
  Sum/1 -> Divide/2  "T_wall - T_fuel"
  Sum1/1 -> Divide1/2  "T_wall - T_ull"
  wet HTC/1 -> Divide/1
  total area/1 -> Abs/1  "dry area"
  Divide/1 -> Qwall_wet/1
  Divide1/1 -> Qwall_dry/1
  dry HTC/1 -> Divide1/1
  Abs/1 -> dry HTC/1

== system ECS_FOS/ECS/FOHX Left Wing/HX_Calcs/Fluid 1 Heat Transfer Calculation/HTC Calc ==
  note: Calculation of secondary fluid heat transfer coefficient using the Longo correlation
  mdot_a : Inport
  A_ca : Inport  Port=2
  T_a : Inport  Port=3
  Constant1 : Constant  Value=alpha1
  Terminator : Terminator
  Terminator1 : Terminator
  Terminator2 : Terminator
  alpha_a : Outport
  wires:
  Constant1/1 -> alpha_a/1
  mdot_a/1 -> Terminator/1
  A_ca/1 -> Terminator1/1
  T_a/1 -> Terminator2/1

== system ECS_FOS/ECS/FOHX Left Wing/HX_Calcs/Fluid 2 Heat Transfer Calculation/HTC Calc ==
  note: Calculation of secondary fluid heat transfer coefficient using the Longo correlation
  mdot_a : Inport
  A_ca : Inport  Port=2
  T_a : Inport  Port=3
  Constant1 : Constant  Value=alpha2
  Terminator : Terminator
  Terminator1 : Terminator
  Terminator2 : Terminator
  alpha_a : Outport
  wires:
  Constant1/1 -> alpha_a/1
  mdot_a/1 -> Terminator/1
  A_ca/1 -> Terminator1/1
  T_a/1 -> Terminator2/1

== system ECS_FOS/ECS/FOHX Right Wing/HX_Calcs/Fluid 1 Heat Transfer Calculation/HTC Calc ==
  note: Calculation of secondary fluid heat transfer coefficient using the Longo correlation
  mdot_a : Inport
  A_ca : Inport  Port=2
  T_a : Inport  Port=3
  Constant1 : Constant  Value=alpha1
  Terminator : Terminator
  Terminator1 : Terminator
  Terminator2 : Terminator
  alpha_a : Outport
  wires:
  T_a/1 -> Terminator2/1
  A_ca/1 -> Terminator1/1
  mdot_a/1 -> Terminator/1
  Constant1/1 -> alpha_a/1

== system ECS_FOS/ECS/FOHX Right Wing/HX_Calcs/Fluid 2 Heat Transfer Calculation/HTC Calc ==
  note: Calculation of secondary fluid heat transfer coefficient using the Longo correlation
  mdot_a : Inport
  A_ca : Inport  Port=2
  T_a : Inport  Port=3
  Constant1 : Constant  Value=alpha2
  Terminator : Terminator
  Terminator1 : Terminator
  Terminator2 : Terminator
  alpha_a : Outport
  wires:
  T_a/1 -> Terminator2/1
  A_ca/1 -> Terminator1/1
  mdot_a/1 -> Terminator/1
  Constant1/1 -> alpha_a/1
